simulink model "LKAS_AutoSave_DF_20220215_0920"  (R2018b)
settings: Solver=FixedStepDiscrete  StartTime=0.0  StopTime=10.0  FixedStep=0.01  RelTol=1e-3
InitFcn:
  | tmpVer = ver('MATLAB');
  | tmpVer = str2num(tmpVer.Version);
  | % -------------------------------------------------------------------
  | %  MATLAB file generated by Simulink.saveVars on 21-Nov-2019 10:06:14
  | %  MATLAB version: 7.13.0.564 (R2011b)
  | % -------------------------------------------------------------------
  | 
  | 
  | SInt16 = Simulink.AliasType;
  | SInt16.Description = 'Num';
  | if (tmpVer > 7.11)
  | 	SInt16.DataScope = 'Auto';
  | end
  | SInt16.HeaderFile = 'Rte_Type.h';
  | SInt16.BaseType = 'int16';
  | 
  | SInt32 = Simulink.AliasType;
  | SInt32.Description = 'Num';
  | if (tmpVer > 7.11)
  | 	SInt32.DataScope = 'Auto';
  | end
  | SInt32.HeaderFile = 'Rte_Type.h';
  | SInt32.BaseType = 'int32';
  | 
  | SInt8 = Simulink.AliasType;
  | SInt8.Description = 'Num';
  | if (tmpVer > 7.11)
  | 	SInt8.DataScope = 'Auto';
  | end
  | SInt8.HeaderFile = 'Rte_Type.h';
  | SInt8.BaseType = 'int8';
  | 
  | T_A_m2_1024_1_u32 = Simulink.NumericType;
  | T_A_m2_1024_1_u32.Description = 'm2 (square meters  (m2))';
  | if (tmpVer > 7.11)
  | 	T_A_m2_1024_1_u32.DataScope = 'Auto';
  | end
  | T_A_m2_1024_1_u32.HeaderFile = 'Rte_Type.h';
  | T_A_m2_1024_1_u32.DataTypeMode = 'Fixed-point: slope and bias scaling';
  | T_A_m2_1024_1_u32.SignednessBool = false;
  | T_A_m2_1024_1_u32.WordLength = 32;
  | T_A_m2_1024_1_u32.FixedExponent = -10;
  | T_A_m2_1024_1_u32.SlopeAdjustmentFactor = 1;
  | T_A_m2_1024_1_u32.Bias = 0;
  | T_A_m2_1024_1_u32.DataTypeOverride = 'Inherit';
  | T_A_m2_1024_1_u32.IsAlias = true;
  | 
  | T_A_m2_65536_1_u16 = Simulink.NumericType;
  | T_A_m2_65536_1_u16.Description = 'm2 (square meters  (m2))';
  | if (tmpVer > 7.11)
  | 	T_A_m2_65536_1_u16.DataScope = 'Auto';
  | end
  | T_A_m2_65536_1_u16.HeaderFile = 'Rte_Type.h';
  | T_A_m2_65536_1_u16.DataTypeMode = 'Fixed-point: slope and bias scaling';
  | T_A_m2_65536_1_u16.SignednessBool = false;
  | T_A_m2_65536_1_u16.WordLength = 16;
  | T_A_m2_65536_1_u16.FixedExponent = -16;
  | T_A_m2_65536_1_u16.SlopeAdjustmentFactor = 1;
  | T_A_m2_65536_1_u16.Bias = 0;
  | T_A_m2_65536_1_u16.DataTypeOverride = 'Inherit';
  | ... (+4647 lines)
StopFcn:
  | clear  T_A_m2_1024_1_u32 T_A_m2_65536_1_u16 T_A_m2_Float32 T_A_mm2_10_1_u16 T_A_mm2_4_1_s16 T_A_mm2_Float32 T_Cnt_Num_10_1_u32 T_Cnt_Num_1_1_s16 T_Cnt_Num_1_1_s32 T_Cnt_Num_1_1_s8 T_Cnt_Num_1_1_u16 T_Cnt_Num_1_1_u32 T_Cnt_Num_1_1_u8 T_E_J_1_1_s32 T_E_J_Float32 T_E_kJ_128_1_s32 T_E_kJ_Float32 T_E_kwh_10_1_u16 T_E_kwh_Float32 T_Epl_kwhpkm_100_1_u16 T_Epl_kwhpkm_Float32 T_F_N_1_1_s16 T_F_N_Float32 T_I_A_1000_1_u16 T_I_A_1048576_1_s32 T_I_A_2048_1_s16 T_I_A_32_1_s16 T_I_A_Float32 T_I_mA_1_1_s16 T_I_mA_32768_128_s16 T_I_mA_Float32 T_J_kgpm2_128_1_u16 T_J_kgpm2_Float32 T_K_NA_1000_1_s16 T_K_NA_100_1_s16 T_K_NA_100_1_u16 T_K_NA_1024_1_s16 T_K_NA_1024_1_u16 T_K_NA_128_1_s16 T_K_NA_128_1_u16 T_K_NA_128_1_u8 T_K_NA_16777216_1_u32 T_K_NA_16_1_s16 T_K_NA_16_1_u16 T_K_NA_16_1_u8 T_K_NA_1_16_u16 T_K_NA_1_1_s16 T_K_NA_1_1_u16 T_K_NA_1_1_u8 T_K_NA_32768_1_s16 T_K_NA_32768_1_u16 T_K_NA_32_1_s8 T_K_NA_4096_1_u16 T_K_NA_4194304_1_s32 T_K_NA_4194304_1_u16 T_K_NA_65536_1_s32 T_K_NA_65536_1_u16 T_K_NA_8192_1_s16 T_K_NA_8_1_s16 T_K_NA_Float32 T_M_Nm_16_1_s16 T_M_Nm_1_1_s16 T_M_Nm_32768_1_s16 T_M_Nm_32_1_s16 T_M_Nm_4_1_s16 T_M_Nm_512_1_s16 T_M_Nm_Float32 T_P_W_1_4_s16 T_P_W_1_8_s16 T_P_W_Float32 T_P_kW_128_1_s16 T_P_kW_1_8_s16 T_P_kW_8_1_s32 T_P_kW_Float32 T_Pct_pct_1024_1_s32 T_Pct_pct_1024_1_u32 T_Pct_pct_10_1_s16 T_Pct_pct_10_1_u32 T_Pct_pct_128_100_s8 T_Pct_pct_1_1_s16 T_Pct_pct_1_4_u8 T_Pct_pct_255_100_u16 T_Pct_pct_255_100_u8 T_Pct_pct_256_1_s16 T_Pct_pct_256_1_u16 T_Pct_pct_65535_100_u16 T_Pct_pct_Float32 T_R_ohm_1024_1_s16 T_R_ohm_32_1_s16 T_R_ohm_Float32 T_TK_K_16_1_s16 T_TK_K_Float32 T_T_degC_10_400_1_u16 T_T_degC_16_1_s16 T_T_degC_1_40_1_u8 T_T_degC_2_80_1_u8 T_T_degC_Float32 T_U_V_1000_1_u16 T_U_V_10_1_u8 T_U_V_200_1_u8 T_U_V_32_1_s16 T_U_V_4096_1_s16 T_U_V_512_1_s16 T_U_V_65535_8_u16 T_U_V_8192_1_u16 T_U_V_Float32 T_U_mV_1_1_s16 T_U_mV_256_20_u16 T_U_mV_Float32 T_V_l_256_1_s16 T_V_l_4096_1_s16 T_V_l_64_1_s16 T_V_l_65535_100_u16 T_V_l_Float32 T_V_ml_128_1_s16 T_V_ml_1_1_s16 T_V_ml_32768_1_s16 T_V_ml_Float32 T_V_ul_32_1_u16 T_V_ul_Float32 T_Vpl_clpkm_512_1_u16 T_Vpl_clpkm_Float32 T_a_kphps_16_1_s16 T_a_kphps_Float32 T_a_mps2_128_1_s16 T_a_mps2_Float32 T_c_MJpkg_256_1_s16 T_c_MJpkg_Float32 T_c_kJpgpK_1024_1_s16 T_c_kJpgpK_Float32 T_c_kJpkgpK_128_1_u16 T_c_kJpkgpK_Float32 T_chrg_Ah_1_1_s16 T_chrg_Ah_1_1_u16 T_chrg_Ah_1_1_u8 T_chrg_Ah_256_1_u16 T_chrg_Ah_4194304_1_s32 T_chrg_Ah_512_1_u16 T_chrg_Ah_8_1_u16 T_chrg_Ah_Float32 T_cmp_NA_100_1_s16 T_cmp_NA_128_1_s16 T_cmp_NA_16_1_s16 T_cmp_NA_32768_1_u16 T_cmp_NA_Float32 T_d2n_rpmps2_4_1_s16 T_d2n_rpmps2_Float32 T_dPct_pctps_16_1_s16 T_dPct_pctps_256_1_s16 T_dPct_pctps_Float32 T_dT_degCps_128_1_s16 T_dT_degCps_Float32 T_dV_lph_1_1_s16 T_dV_lph_Float32 T_dV_lpm_128_1_s16 T_dV_lpm_32_1_s16 T_dV_lpm_Float32 T_dV_lps_1024_1_u16 T_dV_lps_4_1_u16 T_dV_lps_Float32 T_dV_mlps_1024_1_s16 T_dV_mlps_Float32 T_d_BitField16 T_dm_gps_128_1_s16 T_dm_gps_128_1_u16 T_dm_gps_256_1_u16 T_dm_gps_Float32 T_dm_mgps_1_1_s16 T_dm_mgps_Float32 T_dn_rpmps_1_1_s16 T_dn_rpmps_2_1_s16 T_dn_rpmps_Float32 T_dp_Paps_1_1_s16 T_dp_Paps_Float32 T_dp_kPaps_1_1_s16 T_dp_kPaps_8_1_s16 T_dp_kPaps_Float32 T_dphi_degps_128_1_s16 T_dphi_degps_8_1_s16 T_dphi_degps_Float32 T_dr_ps_256_1_s16 T_dr_ps_Float32 T_drho_mgplps_1_2_s16 T_drho_mgplps_Float32 T_e_NA_1_1_u8 T_f_Hz_1_1_u16 T_f_Hz_1_1_u32 T_f_Hz_64_1_u16 T_f_Hz_8_1_s16 T_f_Hz_Float32 T_g_BitField32 T_l_km_16_1_s16 T_l_km_1_1_u16 T_l_km_1_1_u32 T_l_km_Float32 T_l_m_1024_1_s16 T_l_m_16_1_s16 T_l_m_1_1_u32 T_l_m_Float32 T_l_mm_16_1_s16 T_l_mm_1_1_u16 T_l_mm_4096_1_s16 T_l_mm_4_1_u8 T_l_mm_64_1_s16 T_l_mm_Float32 T_m_g_1_1_s16 T_m_g_2048_1_s16 T_m_g_32_1_u16 T_m_g_Float32 T_m_kg_1024_1_s16 T_m_kg_1_1_s16 T_m_kg_1_1_u32 T_m_kg_Float32 T_m_mg_128_1_s16 T_m_mg_32_1_s16 T_m_mg_Float32 T_n_rpm_1_1_s16 T_n_rpm_1_25_u8 T_n_rpm_256_50_u16 T_n_rpm_2_25_u8 T_n_rpm_4_1_u16 T_n_rpm_Float32 T_p_MPa_64_1_s16 T_p_MPa_Float32 T_p_Pa_1_1_s16 T_p_Pa_Float32 T_p_kPa_1_10_u16 T_p_kPa_1_1_s16 T_p_kPa_1_1_u8 T_p_kPa_256_1_u16 T_p_kPa_32_1_u16 T_p_kPa_64_1_s16 T_p_kPa_Float32 T_phi_deg_100_1_s16 T_phi_deg_1024_1_s16 T_phi_deg_128_1_s16 T_phi_deg_1_1_u8 T_phi_deg_256_1_s16 T_phi_deg_2_1_s8 T_phi_deg_32_1_s16 T_phi_deg_512_6_s32 T_phi_deg_Float32 T_phi_rad_2048_1_s16 T_phi_rad_Float32 T_r_NA_1024_1_s16 T_r_NA_1024_1_u16 T_r_NA_16384_1_s16 T_r_NA_16_1_s16 T_r_NA_256_1_s8 T_r_NA_256_1_u16 T_r_NA_32768_1_u16 T_r_NA_32_1_u16 T_r_NA_4096_1_s16 T_r_NA_65535_2_u16 T_r_NA_8192_1_u16 T_r_NA_Float32 T_rho_gpl_8192_1_s16 T_rho_gpl_Float32 T_rho_kgpm3_16_1_s16 T_rho_kgpm3_Float32 T_rho_mgpl_1_1_s16 T_rho_mgpl_64_1_s16 T_rho_mgpl_Float32 T_t_hour_1_1_s16 T_t_hour_Float32 T_t_m_1_1_u16 T_t_m_Float32 T_t_ms_1_1_s16 T_t_ms_1_1_u16 T_t_ms_1_1_u32 T_t_ms_4096_1_s16 T_t_ms_64_1_s16 T_t_ms_Float32 T_t_s_1000_1_s16 T_t_s_100_1_s16 T_t_s_10_1_s16 T_t_s_10_1_u16 T_t_s_1_1_s16 T_t_s_1_1_u16 T_t_s_1_1_u32 T_t_s_Float32 T_t_us_10_1_u32 T_t_us_1_1_s16 T_t_us_1_1_u32 T_t_us_1_4_u16 T_t_us_Float32 T_v_kph_1_1_u8 T_v_kph_64_1_s16 T_v_kph_64_1_u16 T_v_kph_Float32 T_v_mps_256_1_s16 T_v_mps_Float32 T_w_radps_32_1_s16 T_w_radps_Float32 T_y_BitField8 T_y_BitFieldDiagProgress T_y_BitFieldDiagStatus T_y_NA_1_1_u8 SInt16 SInt32 SInt8 T_BOOLEAN UInt16 UInt32 UInt8 s16 s32 s8 u16 u32 u8
model workspace (MAT data in the model file):
  MCOS : class17 (value not decoded)
  MCOS : class17 (value not decoded)
  MCOS : class17 (value not decoded)
  MCOS : class17 (value not decoded)
  MCOS : class17 (value not decoded)
  MCOS : class17 (value not decoded)
  MCOS : class17 (value not decoded)
  MCOS : class17 (value not decoded)
  MCOS : class17 (value not decoded)
  MCOS : class17 (value not decoded)
  MCOS : class17 (value not decoded)
  MCOS : class17 (value not decoded)
  MCOS : class17 (value not decoded)
  MCOS : class17 (value not decoded)
  MCOS : class17 (value not decoded)
  MCOS : class17 (value not decoded)
  MCOS : class17 (value not decoded)
  MCOS : class17 (value not decoded)
  MCOS : class17 (value not decoded)
  MCOS : class17 (value not decoded)
  MCOS : class17 (value not decoded)
  MCOS : class17 (value not decoded)
  MCOS : class17 (value not decoded)
  MCOS : class17 (value not decoded)
  MCOS : class17 (value not decoded)
  MCOS : class17 (value not decoded)
  MCOS : class17 (value not decoded)
  MCOS : class17 (value not decoded)
  MCOS : class17 (value not decoded)
  MCOS : class17 (value not decoded)
  MCOS : class17 (value not decoded)
  MCOS : class17 (value not decoded)
  MCOS : class17 (value not decoded)
  MCOS : class17 (value not decoded)
  MCOS : class17 (value not decoded)
  MCOS : class17 (value not decoded)
  MCOS : class17 (value not decoded)
  MCOS : class17 (value not decoded)
  MCOS : class17 (value not decoded)
  MCOS : class17 (value not decoded)
  MCOS : class17 (value not decoded)
  MCOS : class17 (value not decoded)
  MCOS : class17 (value not decoded)
  MCOS : class17 (value not decoded)
  MCOS : class17 (value not decoded)
  MCOS : class17 (value not decoded)
  MCOS : class17 (value not decoded)
  MCOS : class17 (value not decoded)
  MCOS : class17 (value not decoded)
  MCOS : class17 (value not decoded)
  MCOS : class17 (value not decoded)
  MCOS : class17 (value not decoded)
  MCOS : class17 (value not decoded)
  MCOS : class17 (value not decoded)
  MCOS : class17 (value not decoded)
  MCOS : class17 (value not decoded)
  MCOS : class17 (value not decoded)
  MCOS : class17 (value not decoded)
  MCOS : class17 (value not decoded)
  MCOS : class17 (value not decoded)
  MCOS : class17 (value not decoded)
  MCOS : class17 (value not decoded)
  MCOS : class17 (value not decoded)
  MCOS : class17 (value not decoded)
  MCOS : class17 (value not decoded)
  MCOS : class17 (value not decoded)
  MCOS : class17 (value not decoded)
  MCOS : class17 (value not decoded)
  MCOS : class17 (value not decoded)
  MCOS : class17 (value not decoded)
  MCOS : class17 (value not decoded)
  MCOS : class17 (value not decoded)
  MCOS : class17 (value not decoded)
  MCOS : class17 (value not decoded)
  MCOS : class17 (value not decoded)
  MCOS : class17 (value not decoded)
  MCOS : class17 (value not decoded)
  MCOS : class17 (value not decoded)
  MCOS : class17 (value not decoded)
  MCOS : class17 (value not decoded)
  MCOS : class17 (value not decoded)
  MCOS : class17 (value not decoded)
  MCOS : class17 (value not decoded)
  MCOS : class17 (value not decoded)
  MCOS : class17 (value not decoded)
  MCOS : class17 (value not decoded)
  MCOS : class17 (value not decoded)
  MCOS : class17 (value not decoded)
  MCOS : class17 (value not decoded)
  MCOS : class17 (value not decoded)
  MCOS : class17 (value not decoded)
  MCOS : class17 (value not decoded)
  MCOS : class17 (value not decoded)
  MCOS : class17 (value not decoded)
  MCOS : class17 (value not decoded)
  MCOS : class17 (value not decoded)
  MCOS : class17 (value not decoded)
  MCOS : class17 (value not decoded)
  MCOS : class17 (value not decoded)
  MCOS : class17 (value not decoded)
  MCOS : class17 (value not decoded)
  MCOS : class17 (value not decoded)
undefined symbols (not defined in the file): LKA_CarWidth, LKA_SampleTime, LKA_StrRatio_C, LKA_Veh2CamL_C, LKA_Veh2CamW_C, LKA_WhlBaseL_C, LL_CompHdAg_C, LL_CompSWA_C, LL_CrvtPrvwT_C, LL_DesDvt_C, LL_DvtComp_C, LL_DvtPrvwT_C, LL_DvtSpdDet_vDvtSpdMin_C, LL_HandsOff_ExitTime, LL_HandsOff_TextTime, LL_HandsOff_WarnTime, LL_HdAgExT_C, LL_HdAgPrvwT_C, LL_LAccMax_C, LL_LAccRMax_C, LL_LDW_EarliestWarnLine_C, LL_LDW_LatestWarnLine_C, LL_LDWS_SUPPRESS_HEADING, LL_LFClb_TFC_FfCtlRatio_C, LL_LFClb_TFC_KdBalance_C, LL_LFClb_TFC_KdMaxSWA_C, LL_LFClb_TFC_KdV1_C, LL_LFClb_TFC_KdV2_C, LL_LFClb_TFC_KdVehSpdLwr_C, LL_LFClb_TFC_KdVehSpdUpr_C, LL_LFClb_TFC_Ki_C, LL_LFClb_TFC_KiMaxSWA_C, LL_LFClb_TFC_Kp_C, LL_LFClb_TFC_KpKlat_C, LL_LFClb_TFC_KpV1_C, LL_LFClb_TFC_KpV2_C, LL_LFClb_TFC_KpVehSpdLwr_C, LL_LFClb_TFC_KpVehSpdUpr_C, LL_LFClb_TFC_PrvwT_C, LL_LKA_EarliestWarnLine_C, LL_LKA_LatestWarnLine_C, LL_LKAExPrcs_ExitC0Dvt, LL_LKAExPrcs_ExitC0Swt, LL_LKAExPrcs_tiExitTime1, LL_LKAExPrcs_tiExitTime2, LL_LKAExPrcs_tiExitTime3, LL_LKAS_OUT_OF_CONTROL_LAT_VEL, LL_LKAS_OUT_OF_CONTROL_TTLC, LL_LKASWASyn_M0, LL_LKASWASyn_M1, LL_LKASWASyn_M2, LL_LKASWASyn_M3K, LL_LKASWASyn_SWAaddMax, LL_LKASWASyn_T2, LL_LKASWASyn_tiTrqSwaRtTime, LL_LKASWASyn_tiTrqSwaTime, LL_LKASWASyn_TrqMax, LL_LKASWASyn_TrqSwaAddSwt, LL_LKASWASyn_TrqSwaRateDiff, LL_LSpdCompT_C ... (+43)
libraries: simulink x136, canmsglib x8, dspstat3 x3, simulink_extras x1
(part 13 of 20)

== system LKAS_AutoSave_DF_20220215_0920/LKAS/LL/LLOn/LL State Determination (LLStateDet)/LL State Machine Conditions (LLSMCon)/Activation Condition (ActvC)/EPS Controllability Enable Condition (EPSCtlEC) ==
  EPSCtlEC_bsEPSInfo : Inport
  Bus Selector : BusSelector  OutputSignals=EPS_LKA_State
  Compare To Constant : simulink/Logic and Bit Operations/Compare To Constant  relop===  const=1  OutDataTypeStr=boolean
  Compare To Constant1 : simulink/Logic and Bit Operations/Compare To Constant  relop===  const=3  OutDataTypeStr=boolean
  Data Type Conversion : DataTypeConversion  OutDataTypeStr=uint8
  Logical Operator : Logic  Operator=OR  AllPortsSameDT=off  OutDataTypeStr=boolean
  EPSCtlEC_stEPSCtlEC : Outport
  wires:
  Data Type Conversion/1 -> EPSCtlEC_stEPSCtlEC/1
  Compare To Constant1/1 -> Logical Operator/2
  EPSCtlEC_bsEPSInfo/1 -> Bus Selector/1
  Bus Selector/1 -> Compare To Constant1/1, Compare To Constant/1  "<EPS_LKA_State>"
  Compare To Constant/1 -> Logical Operator/1
  Logical Operator/1 -> Data Type Conversion/1

== system LKAS_AutoSave_DF_20220215_0920/LKAS/LL/LLOn/LL State Determination (LLStateDet)/LL State Machine Conditions (LLSMCon)/Activation Condition (ActvC)/Lane Quality Enable Condition (LaneQlEC) ==
  LaneQlEC_InInfoSyn : Inport
  LaneQlEC_SingleLane_Disable_Swt : Inport  Port=2
  LaneQlEC_stDvtThresActvFlg : Inport  Port=3
  LaneQlEC_stFacmL0Ql : Inport  Port=4
  LaneQlEC_stFacmR0Ql : Inport  Port=5
  Bus Selector : BusSelector  OutputSignals=bsLLSMConClb.DisblCClb.LL_SingleLane_Disable_Swt
  Bus Selector1 : BusSelector  OutputSignals=bsBCMInfo.BCM_Left_Light,bsBCMInfo.BCM_Right_Light
  Compare To Constant : simulink/Logic and Bit Operations/Compare To Constant  relop=>  const=2  OutDataTypeStr=boolean
  Compare To Constant1 : simulink/Logic and Bit Operations/Compare To Constant  relop=>  const=2  OutDataTypeStr=boolean
  Compare To Constant2 : simulink/Logic and Bit Operations/Compare To Constant  relop===  const=2  OutDataTypeStr=boolean
  Compare To Constant3 : simulink/Logic and Bit Operations/Compare To Constant  relop===  const=1  OutDataTypeStr=boolean
  Data Type Conversion : DataTypeConversion  OutDataTypeStr=uint8
  Logical Operator : Logic  Inputs=3  AllPortsSameDT=off  OutDataTypeStr=boolean
  Logical Operator1 : Logic  Inputs=3  AllPortsSameDT=off  OutDataTypeStr=boolean
  Logical Operator2 : Logic  Operator=OR  AllPortsSameDT=off  OutDataTypeStr=boolean
  Logical Operator3 : Logic  Operator=NOT  AllPortsSameDT=off  OutDataTypeStr=boolean
  Logical Operator4 : Logic  Operator=NOT  AllPortsSameDT=off  OutDataTypeStr=boolean
  Logical Operator5 : Logic  Operator=OR  AllPortsSameDT=off  OutDataTypeStr=boolean
  Logical Operator6 : Logic  Operator=NOT  AllPortsSameDT=off  OutDataTypeStr=boolean
  Logical Operator7 : Logic  Operator=OR  AllPortsSameDT=off  OutDataTypeStr=boolean
  LaneQlEC_stLaneQlECFlgLKA : Outport
  wires:
  LaneQlEC_stFacmL0Ql/1 -> Compare To Constant/1
  LaneQlEC_stFacmR0Ql/1 -> Compare To Constant1/1
  Data Type Conversion/1 -> LaneQlEC_stLaneQlECFlgLKA/1
  LaneQlEC_stDvtThresActvFlg/1 -> Compare To Constant3/1, Compare To Constant2/1
  Compare To Constant1/1 -> Logical Operator/2
  Compare To Constant2/1 -> Logical Operator/3
  Compare To Constant3/1 -> Logical Operator1/2
  Compare To Constant/1 -> Logical Operator1/3
  Logical Operator/1 -> Logical Operator2/1
  Logical Operator1/1 -> Logical Operator2/2
  Logical Operator2/1 -> Data Type Conversion/1
  LaneQlEC_SingleLane_Disable_Swt/1 -> Bus Selector/1
  Bus Selector/1 -> Logical Operator6/1  "<LL_SingleLane_Disable_Swt>"
  LaneQlEC_InInfoSyn/1 -> Bus Selector1/1
  Bus Selector1/1 -> Logical Operator3/1  "<BCM_Left_Light>"
  Bus Selector1/2 -> Logical Operator4/1  "<BCM_Right_Light>"
  Logical Operator3/1 -> Logical Operator5/2
  Logical Operator6/1 -> Logical Operator7/1, Logical Operator5/1
  Logical Operator4/1 -> Logical Operator7/2
  Logical Operator7/1 -> Logical Operator/1
  Logical Operator5/1 -> Logical Operator1/1

== system LKAS_AutoSave_DF_20220215_0920/LKAS/LL/LLOn/LL State Determination (LLStateDet)/LL State Machine Conditions (LLSMCon)/Deactivation Condition (DeactvC)/Deactivation Condition Synthesis (DeactvCSyn) ==
  DeactvCSyn_stDACMode : Inport
  DeactvCSyn_stDvtThresActvFlgLDW : Inport  Port=2
  DeactvCSyn_stDvtThresActvFlgLKA : Inport  Port=3
  DvrTkCon_stDvrTkConFlg : Inport  Port=4
  DeactvCSyn_stEPSCFlg : Inport  Port=5
  DeactvCSyn_stExitFlg : Inport  Port=6
  Cast To Single : DataTypeConversion  OutDataTypeStr=uint8
  Cast To Single1 : DataTypeConversion  OutDataTypeStr=uint8
  Default Flag (DflFlg) : Subsystem  TreatAsAtomicUnit=on
  Default Flag (DflFlg)1 : Subsystem  TreatAsAtomicUnit=on
  If : If  NumInputs=2  IfExpression=(u1 ==1|u1==2)& u2 == 0
  If1 : If  NumInputs=4  IfExpression=u1 == 2 & (u3 == 1 | u4 == 1)
  LDW Deactivation Flag (LDWDeactvFlg) : Subsystem  TreatAsAtomicUnit=on
  LKA Deactivation Flag (LKADeactvFlg) : Subsystem  TreatAsAtomicUnit=on
  Logical Operator : Logic  Operator=OR  AllPortsSameDT=off  OutDataTypeStr=boolean
  Merge : Merge
  Merge1 : Merge
  DeactvCSyn_stLDWDeactvCSyn : Outport
  DeactvCSyn_stLKADeactvCSyn : Outport  Port=2
  wires:
  Cast To Single1/1 -> If1/4
  LDW Deactivation Flag (LDWDeactvFlg)/1(Out) -> Merge/1
  If/1 -> LDW Deactivation Flag (LDWDeactvFlg)/Action
  If/2 -> Default Flag (DflFlg)/Action
  DeactvCSyn_stDACMode/1 -> If1/1, If/1
  DeactvCSyn_stDvtThresActvFlgLKA/1 -> If1/2
  Default Flag (DflFlg)/1(Out) -> Merge/2
  If1/2 -> Default Flag (DflFlg)1/Action
  Merge1/1 -> DeactvCSyn_stLKADeactvCSyn/1
  DeactvCSyn_stEPSCFlg/1 -> Logical Operator/2
  DeactvCSyn_stExitFlg/1 -> Cast To Single1/1
  LKA Deactivation Flag (LKADeactvFlg)/1(Out) -> Merge1/1
  Default Flag (DflFlg)1/1(Out) -> Merge1/2
  If1/1 -> LKA Deactivation Flag (LKADeactvFlg)/Action
  Cast To Single/1 -> If1/3
  DvrTkCon_stDvrTkConFlg/1 -> Logical Operator/1
  Logical Operator/1 -> Cast To Single/1
  DeactvCSyn_stDvtThresActvFlgLDW/1 -> If/2
  Merge/1 -> DeactvCSyn_stLDWDeactvCSyn/1

== system LKAS_AutoSave_DF_20220215_0920/LKAS/LL/LLOn/LL State Determination (LLStateDet)/LL State Machine Conditions (LLSMCon)/Deactivation Condition (DeactvC)/Deviation Threshold Condition (DvtThresCon) ==
  DvtThresCon_lLaneWidth : Inport
  DvtThresCon_ILftDvt : Inport  Port=2
  DvtThresCon_IRgtDvt : Inport  Port=3
  DvtThresCon_bsDvtThresClb : Inport  Port=4
  DvtThresCon_InInfoSyn : Inport  Port=5
  Active Lane Calculation (ActLanCalc) : Subsystem
  Bus Selector1 : BusSelector  OutputSignals=bsLaneInfo.bsL0Info.L0_C1,bsVehMovInfo.ESC_VehSpd,bsLaneInfo.bsR0Info.R0_C1
  Deviation Threshold Judgement LDW (DvtThresJdg) : Subsystem
  Deviation Threshold Judgement LKA (DvtThresJdg) : Subsystem
  Divide : Product  Inputs=**  OutDataTypeStr=single
  Divide1 : Product  Inputs=**  OutDataTypeStr=single
  Gain : Gain  Gain=1/3.6  OutDataTypeStr=single
  Saturation1 : Saturate  UpperLimit=2  LowerLimit=-2
      settings: AttributesFormatString="Min = %<LowerLimit>  Max = %<UpperLimit>"
  Saturation5 : Saturate  UpperLimit=2  LowerLimit=-2
      settings: AttributesFormatString="Min = %<LowerLimit>  Max = %<UpperLimit>"
  DvtThresCon_stDvtThresActvFlgLDW : Outport
  DvtThresCon_stDvtThresActvFlgLKA : Outport  Port=2
  wires:
  DvtThresCon_InInfoSyn/1 -> Bus Selector1/1
  Divide1/1 -> Deviation Threshold Judgement LDW (DvtThresJdg)/4(DvtThresJdg_vRgtDvtSpd), Deviation Threshold Judgement LKA (DvtThresJdg)/4(DvtThresJdg_vRgtDvtSpd)
  Divide/1 -> Deviation Threshold Judgement LKA (DvtThresJdg)/3(DvtThresJdg_vLftDvtSpd), Deviation Threshold Judgement LDW (DvtThresJdg)/3(DvtThresJdg_vLftDvtSpd)
  Gain/1 -> Divide1/1, Divide/2
  Bus Selector1/2 -> Gain/1  "<ESC_VehSpd>"
  Bus Selector1/1 -> Divide/1  "<L0_C1>"
  Bus Selector1/3 -> Divide1/2  "<R0_C1>"
  DvtThresCon_lLaneWidth/1 -> Active Lane Calculation (ActLanCalc)/1(ActLanCalc_lLaneWidth)
  DvtThresCon_ILftDvt/1 -> Saturation5/1  "DvtCalc_lLftDvt"
  DvtThresCon_IRgtDvt/1 -> Saturation1/1  "DvtCalc_lRgtDvt"
  Deviation Threshold Judgement LKA (DvtThresJdg)/1(DvtThresJdg_stDvtThresActvFlg) -> DvtThresCon_stDvtThresActvFlgLKA/1  "DvtThresActvFlg"
  Active Lane Calculation (ActLanCalc)/1(ActLanCalc_ActvCClbOut) -> Deviation Threshold Judgement LKA (DvtThresJdg)/5(DvtThresJdg_bsDvtThresClb), Deviation Threshold Judgement LDW (DvtThresJdg)/5(DvtThresJdg_bsDvtThresClb)
  Saturation5/1 -> Deviation Threshold Judgement LDW (DvtThresJdg)/1(DvtThresJdg_lLftDvt), Deviation Threshold Judgement LKA (DvtThresJdg)/1(DvtThresJdg_lLftDvt)
  Saturation1/1 -> Deviation Threshold Judgement LDW (DvtThresJdg)/2(DvtThresJdg_lRgtDvt), Deviation Threshold Judgement LKA (DvtThresJdg)/2(DvtThresJdg_lRgtDvt)
  Deviation Threshold Judgement LDW (DvtThresJdg)/1(DvtThresJdg_stDvtThresActvFlg) -> DvtThresCon_stDvtThresActvFlgLDW/1  "DvtThresActvFlg"
  DvtThresCon_bsDvtThresClb/1 -> Deviation Threshold Judgement LDW (DvtThresJdg)/6(SampleTime), Active Lane Calculation (ActLanCalc)/2(ActLanCalc_Clb)

== system LKAS_AutoSave_DF_20220215_0920/LKAS/LL/LLOn/LL State Determination (LLStateDet)/LL State Machine Conditions (LLSMCon)/Deactivation Condition (DeactvC)/Driver Take Condition (DvrTkCon) ==
  DvrTkCon_crPrvwCrvt : Inport
  DvrTkCon_stActvFlg : Inport  Port=2
  DvrTkCon_bsLLClb : Inport  Port=3
  DvrTkCon_vVehSpd : Inport  Port=4
  DvrTkCon_bsEPSInfo : Inport  Port=5
  Add : Sum
  Bus Selector1 : BusSelector  OutputSignals=EPS_SW_Trq
  Bus Selector2 : BusSelector  OutputSignals=bsLLSMConClb.DisblCClb.LL_MAX_DRIVER_TORQUE_DISABLE,bsLLSMConClb.DisblCClb.LL_TkOvStChk_tiTrqChkT_DEACTV,bsLLSMConClb.DisblCClb.LL_TkOvStChk_tiTDelTime_DEACTV,bsConstantClb.LKA_SampleTime
  Compare To Constant : simulink/Logic and Bit Operations/Compare To Constant  relop=>  const=0  OutDataTypeStr=boolean
  Count : Subsystem
  Count 0.2s : Subsystem
  Logical Operator : Logic  AllPortsSameDT=off  OutDataTypeStr=boolean
  MATLAB Function : MATLAB Function  TreatAsAtomicUnit=on
  Memory : Memory  InheritSampleTime=on
  Time Delay (TDel) : Subsystem
  DvrTkCon_stDvrTkConFlg : Outport
  wires:
  DvrTkCon_bsEPSInfo/1 -> Bus Selector1/1
  DvrTkCon_stActvFlg/1 -> Compare To Constant/1, MATLAB Function/1(stActvFlg)
  Bus Selector1/1 -> MATLAB Function/2(EPSTrq)  "<EPS_SW_Trq>"
  DvrTkCon_vVehSpd/1 -> MATLAB Function/3(VehSpd)
  DvrTkCon_bsLLClb/1 -> Bus Selector2/1
  MATLAB Function/1(stDvrTkConFlg) -> Count 0.2s/Enable
  Count 0.2s/1(Out) -> Time Delay (TDel)/1(TDel_stFlgIn)
  Time Delay (TDel)/1(TDel_stFlgOut) -> Memory/1, DvrTkCon_stDvrTkConFlg/1
  Bus Selector2/4 -> Count 0.2s/1(SampleTime), Time Delay (TDel)/2(SampleTime), Count/1(Input)  "<LKA_SampleTime>"
  DvrTkCon_crPrvwCrvt/1 -> MATLAB Function/5(PrvwCrvt)
  Bus Selector2/1 -> MATLAB Function/4(DisableTrq)  "<LL_MAX_DRIVER_TORQUE_DISABLE>"
  Bus Selector2/2 -> Count 0.2s/2(Sum)  "<LL_TkOvStChk_tiTrqChkT_DEACTV>"
  Add/1 -> Time Delay (TDel)/3(TDel_tiTDel)
  Compare To Constant/1 -> Logical Operator/1
  Logical Operator/1 -> Count/Enable
  Memory/1 -> Logical Operator/2
  Bus Selector2/3 -> Add/1  "<LL_TkOvStChk_tiTDelTime_DEACTV>"
  Count/1(Out) -> Add/2

== system LKAS_AutoSave_DF_20220215_0920/LKAS/LL/LLOn/LL State Determination (LLStateDet)/LL State Machine Conditions (LLSMCon)/Deactivation Condition (DeactvC)/EPS Condition (EPSC) ==
  EPSC_bsLLClb : Inport
  EPSC_bsEPSInfo : Inport  Port=2
  EPSC_bsLLState : Inport  Port=3
  Bus Selector : BusSelector  OutputSignals=EPS_LKA_State
  Bus Selector1 : BusSelector  OutputSignals=LKA_State
  Bus Selector2 : BusSelector  OutputSignals=bsConstantClb.LKA_SampleTime,bsLLSMConClb.DisblCClb.LL_TkOvStChk_tiTDelTime
  Compare To Constant : simulink/Logic and Bit Operations/Compare To Constant  relop=~=  const=3  OutDataTypeStr=boolean
  Compare To Constant1 : simulink/Logic and Bit Operations/Compare To Constant  relop===  const=4  OutDataTypeStr=boolean
  Compare To Constant2 : simulink/Logic and Bit Operations/Compare To Constant  relop===  const=5  OutDataTypeStr=boolean
  Logical Operator : Logic  Operator=OR  AllPortsSameDT=off  OutDataTypeStr=boolean
  Logical Operator1 : Logic  AllPortsSameDT=off  OutDataTypeStr=boolean
  Sum Condition1 : Subsystem  TreatAsAtomicUnit=on
  EPSC_stEPSCFlg : Outport
  wires:
  EPSC_bsEPSInfo/1 -> Bus Selector/1
  Logical Operator1/1 -> EPSC_stEPSCFlg/1
  EPSC_bsLLState/1 -> Bus Selector1/1
  Bus Selector/1 -> Compare To Constant/1  "<EPS_LKA_State>"
  Bus Selector1/1 -> Compare To Constant1/1, Compare To Constant2/1  "<LKA_State>"
  Compare To Constant1/1 -> Logical Operator/1
  Compare To Constant2/1 -> Logical Operator/2
  Compare To Constant/1 -> Logical Operator1/1
  Logical Operator/1 -> Sum Condition1/Enable
  Sum Condition1/1(Out) -> Logical Operator1/2
  Bus Selector2/2 -> Sum Condition1/2(Sum)  "<LL_TkOvStChk_tiTDelTime>"
  EPSC_bsLLClb/1 -> Bus Selector2/1
  Bus Selector2/1 -> Sum Condition1/1(In)  "<LKA_SampleTime>"

== system LKAS_AutoSave_DF_20220215_0920/LKAS/LL/LLOn/LL State Determination (LLStateDet)/LL State Machine Conditions (LLSMCon)/Disable Condition (DisblC)/Disable Condition Synthesis (DisblCSyn) ==
  DisblCSyn_stDACMode : Inport
  DisblCSyn_stVehStateC : Inport  Port=2
  DisblCSyn_stLaneC : Inport  Port=3
  DisblCSyn_stDrvInttC : Inport  Port=4
  DisblCSyn_stLDWOwnC : Inport  Port=5
  DisblCSyn_stLKAOwnC : Inport  Port=6
  DisblCSyn_stLDWAlrmTOut : Inport  Port=7
  Cast To Single : DataTypeConversion  OutDataTypeStr=uint8
  Cast To Single1 : DataTypeConversion  OutDataTypeStr=uint8
  Cast To Single2 : DataTypeConversion  OutDataTypeStr=uint8
  If Action Subsystem1 : Subsystem  TreatAsAtomicUnit=on
  If Action Subsystem2 : Subsystem  TreatAsAtomicUnit=on
  If Action Subsystem3 : Subsystem  TreatAsAtomicUnit=on
  If Action Subsystem4 : Subsystem  TreatAsAtomicUnit=on
  If1 : If  NumInputs=2  IfExpression=(u1 ==1|u1==2)& u2 == 1
  If2 : If  NumInputs=2  IfExpression=u1 == 2 & u2 == 1
  Logical Operator1 : Logic  Operator=OR  AllPortsSameDT=off  OutDataTypeStr=boolean
  Logical Operator2 : Logic  Operator=OR  Inputs=3  AllPortsSameDT=off  OutDataTypeStr=boolean
  Logical Operator3 : Logic  Operator=OR  Inputs=3  AllPortsSameDT=off  OutDataTypeStr=boolean
  Merge1 : Merge
  Merge2 : Merge
  DisblCSyn_stLDWDisblCSyn : Outport
  DisblCSyn_stLKADisblCSyn : Outport  Port=2
  wires:
  DisblCSyn_stVehStateC/1 -> Logical Operator2/1
  DisblCSyn_stLaneC/1 -> Logical Operator2/2
  DisblCSyn_stDrvInttC/1 -> Logical Operator2/3
  DisblCSyn_stLDWOwnC/1 -> Logical Operator3/1
  Logical Operator3/1 -> Cast To Single1/1
  DisblCSyn_stDACMode/1 -> Cast To Single/1
  Logical Operator2/1 -> Logical Operator3/3, Logical Operator1/1
  If Action Subsystem2/1(Out) -> Merge1/1
  If1/1 -> If Action Subsystem2/Action
  If1/2 -> If Action Subsystem4/Action
  Merge1/1 -> DisblCSyn_stLDWDisblCSyn/1
  If Action Subsystem4/1(Out) -> Merge1/2
  DisblCSyn_stLKAOwnC/1 -> Logical Operator1/2
  If Action Subsystem1/1(Out) -> Merge2/1
  If2/1 -> If Action Subsystem1/Action
  If2/2 -> If Action Subsystem3/Action
  If Action Subsystem3/1(Out) -> Merge2/2
  Logical Operator1/1 -> Cast To Single2/1
  Merge2/1 -> DisblCSyn_stLKADisblCSyn/1
  DisblCSyn_stLDWAlrmTOut/1 -> Logical Operator3/2
  Cast To Single/1 -> If2/1, If1/1
  Cast To Single1/1 -> If1/2
  Cast To Single2/1 -> If2/2

== system LKAS_AutoSave_DF_20220215_0920/LKAS/LL/LLOn/LL State Determination (LLStateDet)/LL State Machine Conditions (LLSMCon)/Disable Condition (DisblC)/Driver Intent Condition (DrvInttC) ==
  DrvInttC_bsInInfoSyn : Inport
  DrvInttC_bsLLClb : Inport  Port=2
  DrvInttC_crPrvwCrvt : Inport  Port=3
  Bus Creator : BusCreator  Inputs=3
  Bus Selector : BusSelector  OutputSignals=bsSWAInfo.SW_Angle,bsSWAInfo.SW_Angle_Speed,bsVehMovInfo.ESC_LatAcc,bsVehMovInfo.ESC_LonAcc,bsEPSInfo,bsVehMovInfo.ESC_VehSpd
  Driver Action Condition Synthesis (DrvActnCSyn) : Subsystem  Description=|
      | Block Name: Driver Action Condition Synthesis
      | Ab.: DrvActnCSyn
      | No.: 1.1.1.3.3.5
      | Rev: 0.0.1
      | Update Date: 19-3-26
  Driver Action Detection (DrvActnDet) : Subsystem  Description=|
      | Block Name: Driver Action Detection
      | Ab.: DrvActnDet
      | No.: 1.1.1.3.3.1
      | Rev: 0.0.1
      | Update Date: 19-3-26
  Driver Release Detection (DrvRlsDet) : Subsystem  Description=|
      | Block Name: Driver Release Detection
      | Ab.: DrvRlsDet
      | No.: 1.1.1.2.3.2
      | Rev: 0.0.1
      | Update Date: 19-3-26
  Take-Over Steering Check (TkOvStChk) : Subsystem  Description=|
      | Block Name: Take-Over Steering Check
      | Ab.: TkOvStChk
      | No.: 1.1.1.3.3.4
      | Rev: 0.0.1
      | Update Date: 19-3-26
  DrvInttC_stDrvInttCSyn : Outport
  DrvInttCSyn : Outport  Port=2
  wires:
  Driver Action Condition Synthesis (DrvActnCSyn)/1(DrvActnCSyn_stDrvActnCSyn) -> DrvInttC_stDrvInttCSyn/1  "DRIVER"
  Driver Action Detection (DrvActnDet)/1(DrvActnDet_stTkOvStActvFlg) -> Driver Action Condition Synthesis (DrvActnCSyn)/1(DrvActnCSyn_stTkOvStActvFlg)  "DRIVER_ACT"
  Bus Selector/3 -> Driver Action Detection (DrvActnDet)/3(DrvActnDet_aLAcc)  "<ESC_LatAcc>"
  Bus Selector/4 -> Driver Action Detection (DrvActnDet)/4(DrvActnDet_aFAcc)  "<ESC_LonAcc>"
  Bus Selector/5 -> Take-Over Steering Check (TkOvStChk)/1(TkOvStChk_bsEPSInfo), Driver Release Detection (DrvRlsDet)/1(DrvRlsDet_bsEPSInfo), Driver Action Detection (DrvActnDet)/5(DrvActnDet_bsEPSInfo)  "<bsEPSInfo>"
  Bus Selector/6 -> Take-Over Steering Check (TkOvStChk)/3(TkOvStChk_bsVehSpd)  "<ESC_VehSpd>"
  DrvInttC_bsInInfoSyn/1 -> Bus Selector/1
  DrvInttC_crPrvwCrvt/1 -> Take-Over Steering Check (TkOvStChk)/4(TkOvStChk_crPrvwCrvt)
  Take-Over Steering Check (TkOvStChk)/1(TkOvStChk_stTkOvStChk) -> Driver Action Condition Synthesis (DrvActnCSyn)/3(DrvActnCSyn_stTkOvStChk), Bus Creator/3  "TkOvStChk"
  Driver Release Detection (DrvRlsDet)/1(DrvRlsDet_stDrvRlsDetFlg) -> Driver Action Condition Synthesis (DrvActnCSyn)/2(DrvActnCSyn_stDrvRlsDetFlg), Bus Creator/2  "DRIVER_RELEASE"
  Driver Action Detection (DrvActnDet)/2(DrvActnDet) -> Bus Creator/1  "DrvActnDet"
  Bus Creator/1 -> DrvInttCSyn/1
  Bus Selector/2 -> Driver Action Detection (DrvActnDet)/2(DrvActnDet_dphiSWA_Speed)  "<SW_Angle_Speed>"
  Bus Selector/1 -> Driver Action Detection (DrvActnDet)/1(DrvActnDet_phiSWA)  "<SW_Angle>"
  DrvInttC_bsLLClb/1 -> Driver Release Detection (DrvRlsDet)/2(DrvRlsDet_bsLLClb), Take-Over Steering Check (TkOvStChk)/2(TkOvStChk_bsLLClb), Driver Action Detection (DrvActnDet)/6(DrvInttC_bsLLClb)

== system LKAS_AutoSave_DF_20220215_0920/LKAS/LL/LLOn/LL State Determination (LLStateDet)/LL State Machine Conditions (LLSMCon)/Disable Condition (DisblC)/LDW Alarm Timeout (LDWAlrmTOut) ==
  LDWAlrmTOut_bsLLState : Inport
  LDWAlrmTOut_bsLLClb : Inport  Port=2
  Bus Selector : BusSelector  OutputSignals=LDW_State
  Bus Selector1 : BusSelector  OutputSignals=bsConstantClb.LKA_SampleTime,bsLLSMConClb.DisblCClb.LL_Max_LDWS_Warning_Time
  If Action Subsystem : Subsystem  TreatAsAtomicUnit=on
  If Action Subsystem1 : Subsystem  TreatAsAtomicUnit=on
  Memory : Memory  InheritSampleTime=on
  Merge : Merge
  u1>=3|u1==1&u2==u3 : If  NumInputs=3  IfExpression=u1==4|u1==5&u2==u3
  LDWAlrmTOut_stLDWAlrmTOut : Outport
  wires:
  Bus Selector1/1 -> If Action Subsystem/1(In)  "<LKA_SampleTime>"
  Memory/1 -> u1>=3|u1==1&u2==u3/2
  If Action Subsystem1/1(Out1) -> Merge/2
  u1>=3|u1==1&u2==u3/1 -> If Action Subsystem/Action
  u1>=3|u1==1&u2==u3/2 -> If Action Subsystem1/Action
  If Action Subsystem/1(Out) -> Merge/1
  LDWAlrmTOut_bsLLState/1 -> Bus Selector/1
  Bus Selector/1 -> u1>=3|u1==1&u2==u3/1, u1>=3|u1==1&u2==u3/3, Memory/1  "<LDW_State>"
  LDWAlrmTOut_bsLLClb/1 -> Bus Selector1/1
  Bus Selector1/2 -> If Action Subsystem/2(Sum)  "<LL_Max_LDWS_Warning_Time>"
  Merge/1 -> LDWAlrmTOut_stLDWAlrmTOut/1

== system LKAS_AutoSave_DF_20220215_0920/LKAS/LL/LLOn/LL State Determination (LLStateDet)/LL State Machine Conditions (LLSMCon)/Disable Condition (DisblC)/LDW Own Condition (LDWOwnC) ==
  LDWOwnC_stDACMode : Inport
  LDWOwnC_bsPrDvtInfo : Inport  Port=2
  LDWOwnC_bsLLClb : Inport  Port=3
  Bus Selector : BusSelector  OutputSignals=ILftDvt,IRgtDvt
  Bus Selector1 : BusSelector  OutputSignals=bsLLSMConClb.EnaCClb.LL_LDW_LatestWarnLine_C
  Compare To Constant : simulink/Logic and Bit Operations/Compare To Constant  relop=>=  const=1  OutDataTypeStr=boolean
  Logical Operator : Logic  Operator=OR  AllPortsSameDT=off  OutDataTypeStr=boolean
  Logical Operator1 : Logic  AllPortsSameDT=off  OutDataTypeStr=boolean
  Relational Operator1 : RelationalOperator  Operator=<=  OutDataTypeStr=boolean  RndMeth=Nearest
  Relational Operator2 : RelationalOperator  Operator=<=  OutDataTypeStr=boolean  RndMeth=Nearest
  LDWOwnC_stLDWOwnCSyn : Outport
  wires:
  Logical Operator1/1 -> LDWOwnC_stLDWOwnCSyn/1
  LDWOwnC_bsLLClb/1 -> Bus Selector1/1
  Bus Selector1/1 -> Relational Operator1/2, Relational Operator2/2  "<LL_LDW_LatestWarnLine_C>"
  Bus Selector/2 -> Relational Operator2/1  "<IRgtDvt>"
  Bus Selector/1 -> Relational Operator1/1  "<ILftDvt>"
  LDWOwnC_bsPrDvtInfo/1 -> Bus Selector/1
  Relational Operator2/1 -> Logical Operator/2
  Relational Operator1/1 -> Logical Operator/1
  Logical Operator/1 -> Logical Operator1/2
  Compare To Constant/1 -> Logical Operator1/1
  LDWOwnC_stDACMode/1 -> Compare To Constant/1

== system LKAS_AutoSave_DF_20220215_0920/LKAS/LL/LLOn/LL State Determination (LLStateDet)/LL State Machine Conditions (LLSMCon)/Disable Condition (DisblC)/LKA Own Condition (LKAOwnC) ==
  LKAOwnC_stDACMode : Inport
  LKAOwnC_bsInInfoSyn : Inport  Port=2
  LKAOwnC_bsTTLCInfo : Inport  Port=3
  LKAOwnC_bsLLState : Inport  Port=4
  LKAOwnC_bsLLClb : Inport  Port=5
  LKAOwnC_bsDvtInfo : Inport  Port=6
  Bus Creator : BusCreator  Inputs=3
  Bus Selector : BusSelector  OutputSignals=bsEPSInfo
  Bus Selector1 : BusSelector  OutputSignals=bsLLSMConClb.EnaCClb.LL_LKAS_OUT_OF_CONTROL_LAT_VEL,bsLLSMConClb.EnaCClb.LL_LKA_LatestWarnLine_C,bsLLSMConClb.DisblCClb.LL_MAX_DELAY_EPSSTAR_TIME,bsConstantClb.LKA_SampleTime
  Bus Selector2 : BusSelector  OutputSignals=ILftDvt,IRgtDvt
  EPS Condition (EPSC) : Subsystem  Description=|
      | Block Name: EPS Condition
      | Ab.: EPSC
      | No.: 1.1.1.3.5.3
      | Rev: 0.0.1
      | Update Date: 19-3-26
  LKA Own Condition Synthesis (LKAOwnCSyn) : Subsystem  Description=|
      | Block Name: LKA Own Condition Synthesis
      | Ab.: LKAOwnCSyn
      | No.: 1.1.1.3.5.4
      | Rev: 0.0.1
      | Update Date: 19-3-26
  Vehicle Lateral Speed Condition (VehLSpdC) : Subsystem  Description=|
      | Block Name: Vehicle Lateral Speed Condition
      | Ab.: VehLSpdC
      | No.: 1.1.1.3.5.1
      | Rev: 0.0.1
      | Update Date: 19-3-26
  Vehicle Position Check (VehPosChk) : Subsystem  Description=|
      | Block Name: Vehicle Position Check
      | Ab.: VehPosChk
      | No.: 1.1.1.3.5.2
      | Rev: 0.0.1
      | Update Date: 19-3-26
  LKAOwnC_stLKAOwnCSyn : Outport
  LKAOwnC : Outport  Port=2
  wires:
  LKAOwnC_bsInInfoSyn/1 -> Bus Selector/1
  LKAOwnC_bsLLState/1 -> EPS Condition (EPSC)/4(EPSC_bsLLState)
  LKAOwnC_stDACMode/1 -> LKA Own Condition Synthesis (LKAOwnCSyn)/1(LKAOwnCSyn_stDACMode)
  Bus Selector/1 -> EPS Condition (EPSC)/3(EPSC_bsEPSInfo)  "<bsEPSInfo>"
  LKAOwnC_bsLLClb/1 -> Bus Selector1/1
  Bus Selector1/1 -> Vehicle Lateral Speed Condition (VehLSpdC)/2(VehLSpdC_vVehLSpdMax_C)  "<LL_LKAS_OUT_OF_CONTROL_LAT_VEL>"
  Bus Selector1/2 -> Vehicle Position Check (VehPosChk)/3(VehPosChk_lAlrmLine_C)  "<LL_LKA_LatestWarnLine_C>"
  Bus Selector1/3 -> EPS Condition (EPSC)/1(EPSC_tiDelT_C)  "<LL_MAX_DELAY_EPSSTAR_TIME>"
  LKA Own Condition Synthesis (LKAOwnCSyn)/1(LKAOwnCSyn_stLKAOwnCSyn) -> LKAOwnC_stLKAOwnCSyn/1  "LKAOWN"
  LKAOwnC_bsTTLCInfo/1 -> Vehicle Lateral Speed Condition (VehLSpdC)/1(VehLSpdC_bsTTLC)
  Bus Creator/1 -> LKAOwnC/1
  Vehicle Position Check (VehPosChk)/1(VehPosChk_stVehPosChk) -> LKA Own Condition Synthesis (LKAOwnCSyn)/3(LKAOwnCSyn_stVehPosChk), Bus Creator/2  "LKAOWN_VEHPOS"
  EPS Condition (EPSC)/1(EPSC_stEPSC) -> LKA Own Condition Synthesis (LKAOwnCSyn)/4(LKAOwnCSyn_stEPSCtlEC), Bus Creator/3  "LKAOWN_EPS"
  Vehicle Lateral Speed Condition (VehLSpdC)/1(VehLSpdC_stVehLSpdC) -> Bus Creator/1, LKA Own Condition Synthesis (LKAOwnCSyn)/2(LKAOwnCSyn_stVehLSpdC)  "LKAOWN_VEHLATSPEED"
  LKAOwnC_bsDvtInfo/1 -> Bus Selector2/1
  Bus Selector2/1 -> Vehicle Position Check (VehPosChk)/1(VehPosChk_lLftDvt)  "<ILftDvt>"
  Bus Selector2/2 -> Vehicle Position Check (VehPosChk)/2(VehPosChk_lRgtDvt)  "<IRgtDvt>"
  Bus Selector1/4 -> EPS Condition (EPSC)/2(EPSC_tiLKA_SampleTime)  "<LKA_SampleTime>"

== system LKAS_AutoSave_DF_20220215_0920/LKAS/LL/LLOn/LL State Determination (LLStateDet)/LL State Machine Conditions (LLSMCon)/Disable Condition (DisblC)/Lane Condition (LaneC) ==
  LaneC_bsInInfoSyn : Inport
  LaneC_LaneWidth : Inport  Port=2
  LaneC_crPrvwCrvt : Inport  Port=3
  LaneC_bsLLClb : Inport  Port=4
  Bus Creator : BusCreator  Inputs=4
  Bus Selector : BusSelector  OutputSignals=bsLaneInfo.bsL0Info.L0_Q,bsLaneInfo.bsR0Info.R0_Q,bsLaneInfo.bsL0Info.L0_C1,bsLaneInfo.bsR0Info.R0_C1
  Bus Selector1 : BusSelector  OutputSignals=bsLLSMConClb.DisblCClb.LL_MAX_LANE_WIDTH_DISABLE,bsLLSMConClb.DisblCClb.LL_MIN_LANE_WIDTH_DISABLE,bsLLSMConClb.DisblCClb.LL_MAX_SYSTEM_CURVATURE_DISABLE
  Lane C1 Detection (LaneC1Det) : Subsystem  Description=|
      | Block Name: Lane Width Detection
      | Ab.: LaneWDet
      | No.: 1.1.1.3.2.2
      | Rev: 0.0.1
      | Update Date: 19-3-26
  Lane Condition Synthesis (LaneCSyn) : Subsystem  Description=|
      | Block Name: Lane Condition Synthesis
      | Ab.: LaneCSyn
      | No.: 1.1.1.3.2.4
      | Rev: 0.0.1
      | Update Date: 19-3-26
  Lane Curvature Detection (LaneCrvtDet) : Subsystem  Description=|
      | Block Name: Lane Curvature Detection
      | Ab.: LaneCrvtDet
      | No.: 1.1.1.3.2.3
      | Rev: 0.0.1
      | Update Date: 19-3-26
  Lane Quality Disable Condition (LaneQlDC) : Subsystem  Description=|
      | Block Name: Lane Quality Disable Condition
      | Ab.: LaneQlDC
      | No.: 1.1.1.3.2.1
      | Rev: 0.0.1
      | Update Date: 19-3-26
  Lane Width Detection (LaneWDet) : Subsystem  Description=|
      | Block Name: Lane Width Detection
      | Ab.: LaneWDet
      | No.: 1.1.1.3.2.2
      | Rev: 0.0.1
      | Update Date: 19-3-26
  LaneC_stLanCSyn : Outport
  LanCSyn : Outport  Port=2
  wires:
  LaneC_bsInInfoSyn/1 -> Bus Selector/1
  Bus Selector/1 -> Lane Quality Disable Condition (LaneQlDC)/1(LaneQlDC_stFacmL0Ql)  "<L0_Q>"
  Bus Selector/2 -> Lane Quality Disable Condition (LaneQlDC)/2(LaneQlDC_stFacmR0Ql)  "<R0_Q>"
  Lane Condition Synthesis (LaneCSyn)/1(LaneCSyn_stLaneCSyn) -> LaneC_stLanCSyn/1  "LANE"
  Lane Width Detection (LaneWDet)/1(LaneWDet_stLaneWDetFlg) -> Bus Creator/2, Lane Condition Synthesis (LaneCSyn)/2(LaneCSyn_stLaneWDetFlg)  "LANE_WIDTH"
  Bus Selector1/1 -> Lane Width Detection (LaneWDet)/2(LaneWDet_lLaneWMax)  "<LL_MAX_LANE_WIDTH_DISABLE>"
  Bus Selector1/2 -> Lane Width Detection (LaneWDet)/3(LaneWDet_lLaneWMin)  "<LL_MIN_LANE_WIDTH_DISABLE>"
  LaneC_bsLLClb/1 -> Bus Selector1/1
  Bus Selector1/3 -> Lane Curvature Detection (LaneCrvtDet)/2(LaneCrvtDet_crLaneCrvtMax_C)  "<LL_MAX_SYSTEM_CURVATURE_DISABLE>"
  LaneC_crPrvwCrvt/1 -> Lane Curvature Detection (LaneCrvtDet)/1(LaneCrvtDet_crPrvwCrvt)
  Bus Selector/3 -> Lane C1 Detection (LaneC1Det)/1(LaneWDet_facmL0C1)  "<L0_C1>"
  Bus Selector/4 -> Lane C1 Detection (LaneC1Det)/2(LaneWDet_facmR0C1)  "<R0_C1>"
  LaneC_LaneWidth/1 -> Lane Width Detection (LaneWDet)/1(LaneWDet_LaneWidth)
  Lane C1 Detection (LaneC1Det)/1(LaneC1Det_stLaneC1DetFlg) -> Bus Creator/4, Lane Condition Synthesis (LaneCSyn)/4(LaneCSyn_stLaneC1DetFlg)  "LANE_C1"
  Lane Quality Disable Condition (LaneQlDC)/1(LaneQlDC_stLaneQlDCFlg) -> Lane Condition Synthesis (LaneCSyn)/1(LaneCSyn_stLaneQlECFlg), Bus Creator/1  "LANE_Q"
  Bus Creator/1 -> LanCSyn/1
  Lane Curvature Detection (LaneCrvtDet)/1(LaneCrvtDet_stLaneCrvtDetFlg) -> Lane Condition Synthesis (LaneCSyn)/3(LaneCSyn_stLaneCrvtDetFlg), Bus Creator/3  "LANE_CURVAT"

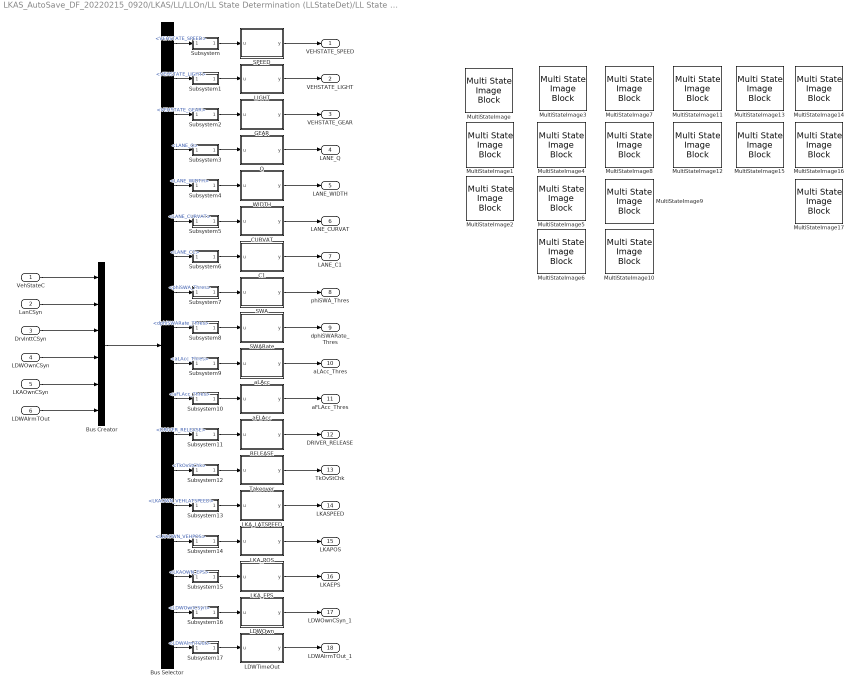
== system LKAS_AutoSave_DF_20220215_0920/LKAS/LL/LLOn/LL State Determination (LLStateDet)/LL State Machine Conditions (LLSMCon)/Disable Condition (DisblC)/Subsystem ==
  VehStateC : Inport
  LanCSyn : Inport  Port=2
  DrvInttCSyn : Inport  Port=3
  LDWOwnCSyn : Inport  Port=4
  LKAOwnCSyn : Inport  Port=5
  LDWAlrmTOut : Inport  Port=6
  Bus Creator : BusCreator  Inputs=6
  Bus Selector : BusSelector  OutputSignals=VehStateC.VEHSTATE_SPEED,VehStateC.VEHSTATE_LIGHT,VehStateC.VEHSTATE_GEAR,LaneCSyn.LANE_Q,LaneCSyn.LANE_WIDTH,LaneCSyn.LANE_CURVAT,LaneCSyn.LANE_C1,DrvInttCSyn.DrvActnDet.phiSWA_Thres,DrvInttCSyn.DrvActnDet.dphiSWARate_Thres,DrvInttCSyn.DrvActnDet.aLAcc_Thres,DrvInttCSyn.DrvActnDet.aFLAcc_Thres,DrvInttCSyn.DRIVER_RELEASE,DrvInttCSyn.TkOvStChk,LKAOwnSyn.LKAOWN_VEHLATSPEED,LKAOwnSyn.LKAOWN_VEHPOS,LKAOwnSyn.LKAOWN_EPS,LDWOwnCSyn,LDWAlrmTOut
  C1 : MATLAB Function  TreatAsAtomicUnit=on
  CURVAT : MATLAB Function  TreatAsAtomicUnit=on
  GEAR : MATLAB Function  TreatAsAtomicUnit=on
  LDWOwn : MATLAB Function  TreatAsAtomicUnit=on
  LDWTimeOut : MATLAB Function  TreatAsAtomicUnit=on
  LIGHT : MATLAB Function  TreatAsAtomicUnit=on
  LKA_EPS : MATLAB Function  TreatAsAtomicUnit=on
  LKA_LATSPEED : MATLAB Function  TreatAsAtomicUnit=on
  LKA_POS : MATLAB Function  TreatAsAtomicUnit=on
  MultiStateImage : MultiStateImageBlock  WebBlockId=3458
  MultiStateImage1 : MultiStateImageBlock  WebBlockId=3459
  MultiStateImage10 : MultiStateImageBlock  WebBlockId=3460
  MultiStateImage11 : MultiStateImageBlock  WebBlockId=3461
  MultiStateImage12 : MultiStateImageBlock  WebBlockId=3462
  MultiStateImage13 : MultiStateImageBlock  WebBlockId=3463
  MultiStateImage14 : MultiStateImageBlock  WebBlockId=3464
  MultiStateImage15 : MultiStateImageBlock  WebBlockId=3465
  MultiStateImage16 : MultiStateImageBlock  WebBlockId=3466
  MultiStateImage17 : MultiStateImageBlock  WebBlockId=3467
  MultiStateImage2 : MultiStateImageBlock  WebBlockId=3468
  MultiStateImage3 : MultiStateImageBlock  WebBlockId=3469
  MultiStateImage4 : MultiStateImageBlock  WebBlockId=3470
  MultiStateImage5 : MultiStateImageBlock  WebBlockId=3471
  MultiStateImage6 : MultiStateImageBlock  WebBlockId=3472
  MultiStateImage7 : MultiStateImageBlock  WebBlockId=3473
  MultiStateImage8 : MultiStateImageBlock  WebBlockId=3474
  MultiStateImage9 : MultiStateImageBlock  WebBlockId=3475
  Q : MATLAB Function  TreatAsAtomicUnit=on
  RELEASE : MATLAB Function  TreatAsAtomicUnit=on
  SPEED : MATLAB Function  TreatAsAtomicUnit=on
  SWA : MATLAB Function  TreatAsAtomicUnit=on
  SWARate : MATLAB Function  TreatAsAtomicUnit=on
  Subsystem : Subsystem
  Subsystem1 : Subsystem
  Subsystem10 : Subsystem
  Subsystem11 : Subsystem
  Subsystem12 : Subsystem
  Subsystem13 : Subsystem
  Subsystem14 : Subsystem
  Subsystem15 : Subsystem
  Subsystem16 : Subsystem
  Subsystem17 : Subsystem
  Subsystem2 : Subsystem
  Subsystem3 : Subsystem
  Subsystem4 : Subsystem
  Subsystem5 : Subsystem
  Subsystem6 : Subsystem
  Subsystem7 : Subsystem
  Subsystem8 : Subsystem
  Subsystem9 : Subsystem
  Takeover : MATLAB Function  TreatAsAtomicUnit=on
  WIDTH : MATLAB Function  TreatAsAtomicUnit=on
  aFLAcc : MATLAB Function  TreatAsAtomicUnit=on
  aLAcc : MATLAB Function  TreatAsAtomicUnit=on
  VEHSTATE_SPEED : Outport
  VEHSTATE_LIGHT : Outport  Port=2
  VEHSTATE_GEAR : Outport  Port=3
  LANE_Q : Outport  Port=4
  LANE_WIDTH : Outport  Port=5
  LANE_CURVAT : Outport  Port=6
  LANE_C1 : Outport  Port=7
  phiSWA_Thres : Outport  Port=8
  dphiSWARate_Thres : Outport  Port=9
  aLAcc_Thres : Outport  Port=10
  aFLAcc_Thres : Outport  Port=11
  DRIVER_RELEASE : Outport  Port=12
  TkOvStChk : Outport  Port=13
  LKASPEED : Outport  Port=14
  LKAPOS : Outport  Port=15
  LKAEPS : Outport  Port=16
  LDWOwnCSyn_1 : Outport  Port=17
  LDWAlrmTOut_1 : Outport  Port=18
  wires:
  Bus Selector/13 -> Subsystem12/1(in1)  "<TkOvStChk>"
  Bus Selector/8 -> Subsystem7/1(in1)  "<phiSWA_Thres>"
  LKAOwnCSyn/1 -> Bus Creator/5
  Bus Selector/17 -> Subsystem16/1(in1)  "<LDWOwnCSyn>"
  Bus Creator/1 -> Bus Selector/1
  VehStateC/1 -> Bus Creator/1
  Bus Selector/4 -> Subsystem3/1(in1)  "<LANE_Q>"
  Bus Selector/18 -> Subsystem17/1(in1)  "<LDWAlrmTOut>"
  LKA_POS/1(y) -> LKAPOS/1
  LDWOwn/1(y) -> LDWOwnCSyn_1/1
  Bus Selector/15 -> Subsystem14/1(in1)  "<LKAOWN_VEHPOS>"
  Bus Selector/11 -> Subsystem10/1(in1)  "<aFLAcc_Thres>"
  Bus Selector/10 -> Subsystem9/1(in1)  "<aLAcc_Thres>"
  Bus Selector/12 -> Subsystem11/1(in1)  "<DRIVER_RELEASE>"
  CURVAT/1(y) -> LANE_CURVAT/1
  Q/1(y) -> LANE_Q/1
  Bus Selector/2 -> Subsystem1/1(in1)  "<VEHSTATE_LIGHT>"
  Bus Selector/9 -> Subsystem8/1(in1)  "<dphiSWARate_Thres>"
  Bus Selector/7 -> Subsystem6/1(in1)  "<LANE_C1>"
  Takeover/1(y) -> TkOvStChk/1
  LanCSyn/1 -> Bus Creator/2
  C1/1(y) -> LANE_C1/1
  Bus Selector/5 -> Subsystem4/1(in1)  "<LANE_WIDTH>"
  DrvInttCSyn/1 -> Bus Creator/3
  LDWOwnCSyn/1 -> Bus Creator/4
  Bus Selector/3 -> Subsystem2/1(in1)  "<VEHSTATE_GEAR>"
  SWARate/1(y) -> dphiSWARate_Thres/1
  RELEASE/1(y) -> DRIVER_RELEASE/1
  Bus Selector/6 -> Subsystem5/1(in1)  "<LANE_CURVAT>"
  LDWAlrmTOut/1 -> Bus Creator/6
  aFLAcc/1(y) -> aFLAcc_Thres/1
  SWA/1(y) -> phiSWA_Thres/1
  LDWTimeOut/1(y) -> LDWAlrmTOut_1/1
  WIDTH/1(y) -> LANE_WIDTH/1
  aLAcc/1(y) -> aLAcc_Thres/1
  GEAR/1(y) -> VEHSTATE_GEAR/1
  LIGHT/1(y) -> VEHSTATE_LIGHT/1
  SPEED/1(y) -> VEHSTATE_SPEED/1
  Bus Selector/1 -> Subsystem/1(in1)  "<VEHSTATE_SPEED>"
  Subsystem/1(Out1) -> SPEED/1(u)
  Subsystem1/1(Out1) -> LIGHT/1(u)
  Subsystem2/1(Out1) -> GEAR/1(u)
  Subsystem3/1(Out1) -> Q/1(u)
  Subsystem4/1(Out1) -> WIDTH/1(u)
  Subsystem5/1(Out1) -> CURVAT/1(u)
  Subsystem6/1(Out1) -> C1/1(u)
  Subsystem7/1(Out1) -> SWA/1(u)
  Subsystem8/1(Out1) -> SWARate/1(u)
  Subsystem9/1(Out1) -> aLAcc/1(u)
  Subsystem10/1(Out1) -> aFLAcc/1(u)
  Subsystem12/1(Out1) -> Takeover/1(u)
  Subsystem11/1(Out1) -> RELEASE/1(u)
  Subsystem16/1(Out1) -> LDWOwn/1(u)
  Subsystem14/1(Out1) -> LKA_POS/1(u)
  Subsystem17/1(Out1) -> LDWTimeOut/1(u)
  LKA_LATSPEED/1(y) -> LKASPEED/1
  Subsystem13/1(Out1) -> LKA_LATSPEED/1(u)
  Bus Selector/14 -> Subsystem13/1(in1)  "<LKAOWN_VEHLATSPEED>"
  LKA_EPS/1(y) -> LKAEPS/1
  Subsystem15/1(Out1) -> LKA_EPS/1(u)
  Bus Selector/16 -> Subsystem15/1(in1)  "<LKAOWN_EPS>"

== system LKAS_AutoSave_DF_20220215_0920/LKAS/LL/LLOn/LL State Determination (LLStateDet)/LL State Machine Conditions (LLSMCon)/Disable Condition (DisblC)/Subsystem1 ==
  VehStateC : Inport
  LanCSyn : Inport  Port=2
  DrvInttCSyn : Inport  Port=3
  LDWOwnCSyn : Inport  Port=4
  LKAOwnCSyn : Inport  Port=5
  LDWAlrmTOut : Inport  Port=6
  Bus Creator : BusCreator  Inputs=6
  Bus Selector : BusSelector  OutputSignals=VehStateC.VEHSTATE_SPEED,VehStateC.VEHSTATE_LIGHT,VehStateC.VEHSTATE_GEAR,LaneCSyn.LANE_Q,LaneCSyn.LANE_WIDTH,LaneCSyn.LANE_CURVAT,LaneCSyn.LANE_C1,DrvInttCSyn.DrvActnDet.phiSWA_Thres,DrvInttCSyn.DrvActnDet.dphiSWARate_Thres,DrvInttCSyn.DrvActnDet.aLAcc_Thres,DrvInttCSyn.DrvActnDet.aFLAcc_Thres,DrvInttCSyn.DRIVER_RELEASE,DrvInttCSyn.TkOvStChk,LKAOwnSyn.LKAOWN_VEHLATSPEED,LKAOwnSyn.LKAOWN_VEHPOS,LKAOwnSyn.LKAOWN_EPS,LDWOwnCSyn,LDWAlrmTOut
  Disable Reason : MATLAB Function  TreatAsAtomicUnit=on
  Mux : Mux  Inputs=18
  DisableReason : Outport
  wires:
  Bus Selector/13 -> Mux/13  "<TkOvStChk>"
  Bus Selector/8 -> Mux/8  "<phiSWA_Thres>"
  LKAOwnCSyn/1 -> Bus Creator/5
  Bus Selector/17 -> Mux/17  "<LDWOwnCSyn>"
  Bus Creator/1 -> Bus Selector/1
  VehStateC/1 -> Bus Creator/1
  Bus Selector/4 -> Mux/4  "<LANE_Q>"
  Bus Selector/18 -> Mux/18  "<LDWAlrmTOut>"
  Bus Selector/15 -> Mux/15  "<LKAOWN_VEHPOS>"
  Bus Selector/11 -> Mux/11  "<aFLAcc_Thres>"
  Bus Selector/10 -> Mux/10  "<aLAcc_Thres>"
  Bus Selector/12 -> Mux/12  "<DRIVER_RELEASE>"
  Bus Selector/2 -> Mux/2  "<VEHSTATE_LIGHT>"
  Bus Selector/9 -> Mux/9  "<dphiSWARate_Thres>"
  Bus Selector/7 -> Mux/7  "<LANE_C1>"
  LanCSyn/1 -> Bus Creator/2
  Bus Selector/5 -> Mux/5  "<LANE_WIDTH>"
  DrvInttCSyn/1 -> Bus Creator/3
  LDWOwnCSyn/1 -> Bus Creator/4
  Bus Selector/3 -> Mux/3  "<VEHSTATE_GEAR>"
  Bus Selector/6 -> Mux/6  "<LANE_CURVAT>"
  LDWAlrmTOut/1 -> Bus Creator/6
  Bus Selector/1 -> Mux/1  "<VEHSTATE_SPEED>"
  Bus Selector/14 -> Mux/14  "<LKAOWN_VEHLATSPEED>"
  Bus Selector/16 -> Mux/16  "<LKAOWN_EPS>"
  Mux/1 -> Disable Reason/1(u)
  Disable Reason/1(y) -> DisableReason/1
